simulink model "W06_Tiny_Town_cs"  (R2019a)
settings: Solver=ode5  StartTime=0.0  StopTime=inf  FixedStep=1/20  RelTol=1e-3
PreLoadFcn:
  | mbxruntime.callbacks.PreLoadFcn(bdroot);
PostLoadFcn:
  | mbxruntime.callbacks.PostLoadFcn(bdroot);
InitFcn:
  | mbxruntime.callbacks.InitFcn(bdroot);
StartFcn:
  | mbxruntime.callbacks.StartFcn(bdroot);
StopFcn:
  | mbxruntime.callbacks.StopFcn(bdroot);
model workspace: external: MAT-File .\W06_Tiny_Town_cs_hws.mat (data not in the file)
undefined symbols (not defined in the file or in its folder): DiscIntNeverNeededParam, InitImageOutputDir, mbxruntime, tabledata, W06_Tiny_Town_cs_0347f368afc477f7, W06_Tiny_Town_cs_06d739b3240d4bd1, W06_Tiny_Town_cs_0f8ec0220805dc92, W06_Tiny_Town_cs_158eea2914cd8c14, W06_Tiny_Town_cs_18b17a0c58606dc8, W06_Tiny_Town_cs_19806d8538d6bb90, W06_Tiny_Town_cs_1ceb610c831ebc6c, W06_Tiny_Town_cs_24c71a941f2399ee, W06_Tiny_Town_cs_28d17e17e50ff375, W06_Tiny_Town_cs_29e44574efa0e72f, W06_Tiny_Town_cs_2ebfd9727ae5049f, W06_Tiny_Town_cs_3b9dd96920beca23, W06_Tiny_Town_cs_4a5ba1a10aa72aa4, W06_Tiny_Town_cs_4b7992cae6b11fea, W06_Tiny_Town_cs_4ce1089559374df3, W06_Tiny_Town_cs_4f1eca6f5670696f, W06_Tiny_Town_cs_56de7514e81a64a4, W06_Tiny_Town_cs_5815099e4ab8d5b1, W06_Tiny_Town_cs_59a193f7803a15f8, W06_Tiny_Town_cs_5a93c0b4041e538b, W06_Tiny_Town_cs_5e22ff2291c0d8f8, W06_Tiny_Town_cs_664a4c8dcb6e1d77, W06_Tiny_Town_cs_66e74ff0a825ce8c, W06_Tiny_Town_cs_6f6fc115e33636b9, W06_Tiny_Town_cs_762b24f74e6359cd, W06_Tiny_Town_cs_7e7dfe0ad6d20cde, W06_Tiny_Town_cs_8dbb769f58f1ae22, W06_Tiny_Town_cs_9732a70429881892, W06_Tiny_Town_cs_97e2037932c1d396, W06_Tiny_Town_cs_99e9b9fe56cd6c11, W06_Tiny_Town_cs_9d4b19fadf9db3f5, W06_Tiny_Town_cs_9e5d5712939b904c, W06_Tiny_Town_cs_9fe5ad465f6cdbf3, W06_Tiny_Town_cs_a263437ac60b94d3, W06_Tiny_Town_cs_a313ed4746bdbf42, W06_Tiny_Town_cs_a3bc7bd64557c06d, W06_Tiny_Town_cs_af25170a5cd54ac4, W06_Tiny_Town_cs_b0bfde99f178c69e, W06_Tiny_Town_cs_b828188f0394b7ed, W06_Tiny_Town_cs_b8ac5a8063403724, W06_Tiny_Town_cs_c0c1ce03c301d04b, W06_Tiny_Town_cs_c5d7b9713d9c4410, W06_Tiny_Town_cs_cce5d3f0bd4fe0dd, W06_Tiny_Town_cs_d4161cd6ae7b274e, W06_Tiny_Town_cs_d7f1a2863608ebc5, W06_Tiny_Town_cs_e07aed9c56d02b7c, W06_Tiny_Town_cs_e4fcf49468faab60, W06_Tiny_Town_cs_e81ada3a1b2b4b0f, W06_Tiny_Town_cs_f328760c8f041e3e, W06_Tiny_Town_cs_fbbe35eb7fc27d63, W06_Tiny_Town_cs_fe7173e9daa72ca4, W06_Tiny_Town_cs_Female_Regular_1_Path_pathUniqueID, W06_Tiny_Town_cs_Ford_Focus_Stationwagon_2_Path_pathUniqueID, W06_Tiny_Town_cs_Nissan_Cabstar_Boxtruck_1_Path_pathUniqueID
libraries: PreScanSimulinkLibrary x16, adeye_lib x14, simulink x4, simulink_extras x3, PreScanUsefulBlocks x1
(part 1 of 7)
CloseFcn:
  | mbxruntime.callbacks.CloseFcn(bdroot);
settings Model: Creator=PRESCAN  LastModifiedBy=adeye
settings DataIOCC: LimitDataPoints=on  SaveFormat=Array  SignalLoggingSaveFormat=ModelDataLogs  ReturnWorkspaceOutputs=off
settings OptimizationCC: DefaultParameterBehavior=Inlined  ExpressionDepthLimit=2147483647  InitFltsAndDblsToZero=on  LifeSpan=inf
settings DebuggingCC: SaveWithParameterizedLinksMsg=none  UnderspecifiedInitializationDetection=Classic  MergeDetectMultiDrivingBlocksExec=none  SignalResolutionControl=TryResolveAllWithWarning  MultiTaskDSMMsg=warning  MultiTaskCondExecSysMsg=none  FcnCallInpInsideContextMsg=warning  StateNameClashWarn=warning  SFUnexpectedBacktrackingDiag=warning  SFNoUnconditionalDefaultTransitionDiag=warning  SFExecutionAtInitializationDiag=none  ArithmeticOperatorsInVariantConditions=warning
settings HardwareCC: ProdBitPerPointer=32  ProdBitPerSizeT=32  ProdBitPerPtrDiffT=32  ProdLargestAtomicFloat=None  ProdIntDivRoundTo=Undefined  ProdEndianess=Unspecified  ProdWordSize=32  ProdHWDeviceType=32-bit Generic
settings ModelReferenceCC: UpdateModelReferenceTargets=IfOutOfDate  PropagateSignalLabelsOutOfModel=off
settings SFSimCC: SimUseLocalCustomCode=off  SimParseCustomCode=off
settings SFSimCC: SimCustomHeaderCode=|
  | #include "prescan.h"
  | #include "prescan_platform.h"
  | #include "prescan_aimsunturnindicatorsetter_data.h"
settings RTWCC: RTWUseLocalCustomCode=off
settings CodeAppCC: StateflowObjectComments=on
settings GRTTargetCC: TargetFcnLib=ansi_tfl_tmw.mat  TargetLangStandard=C89/C90 (ANSI)  GeneratePreprocessorConditionals=Disable all  CombineOutputUpdateFcns=off  GRTInterface=on
settings ConfigComp: CovMetricSettings=dw  CovHtmlReporting=on  CovSaveCumulativeToWorkspaceVar=on  CovSaveSingleToWorkspaceVar=on  CovExternalEMLEnable=off  CovSFcnEnable=off

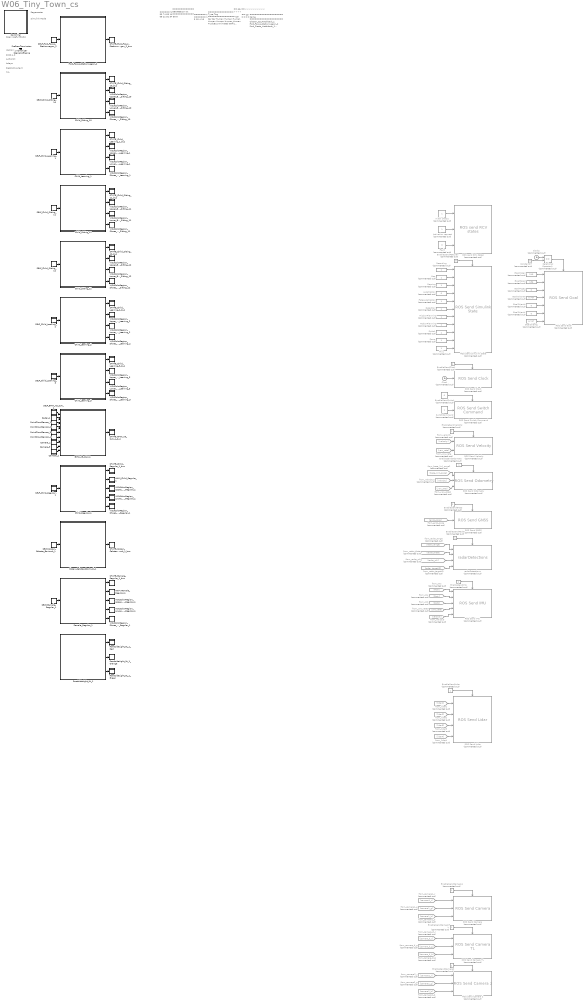
== system W06_Tiny_Town_cs ==
  note: Regenerate
  note: Simulink Mode
  note: Open Useful Blocks
  note: 2020.4.0
  note: Version:
  note: Author(s):
  note: Adeye
  note: Descriptive text:
  note: N.A.
  note: ======
      | Num ID
      | ======
      | 53
      | 74
      | 83
      | 101
      | 102
      | 103
      | 104
      | 67
      | 68
      | 22
      | 52
      | 54
      | 58
      | 8
  note: =============
      | OBU-Beacon ID
      | =============
  note: =======
      | Type ID
      | =======
      | 1
      | 1
      | 1
      | 4
      | 4
      | 4
      | 4
      | 4
      | 4
      | 4
      | 3
      | 15
      | 4
      | 15
  note: ================
      | Type Tag
      | ================
      | Car
      | Car
      | Car
      | Human
      | Human
      | Human
      | Human
      | Human
      | Human
      | Human
      | Truck\Bus
      | Animated traffic sign
      | Human
      | Animated traffic sign
  note: ==
      | SD
      | ==
      | Y
      | Y
      | Y
      | Y
      | Y
      | Y
      | Y
      | Y
      | Y
      | Y
      | Y
      | Y
      | Y
      | Y
  note: ==
      | CD
      | ==
      | N
      | N
      | N
      | N
      | N
      | N
      | N
      | N
      | N
      | N
      | N
      | N
      | N
      | N
  note: ====================
      | Name
      | ====================
      | Citroen_C3_Hatchback_1
      | Ford_Focus_Stationwagon_2
      | Ford_Fiesta_Hatchback_1
      | Child_Sitting_10
      | Child_Leaning_1
      | Child_Sitting_11
      | Child_Sitting_12
      | Child_Leaning_2
      | Child_Leaning_3
      | Child_Regular_1
      | Nissan_Cabstar_Boxtruck_1
      | PedestrianSignal_JP_1
      | Female_Regular_1
      | RoadsideLight_NL_1
  ANIM_Child_Regular_1 : Subsystem  Tag=actuator/AnimationOutport  Priority=0  LoadFcn=load('PreScanAnimActuatorData.mat')  mask(PreScan Sink Block: State Animation){}
      mask help: The Human Animation port allows the human to walk, run or bend
      settings: OpenFcn=open_system([gcb '/Actuator'],'mask')
      mask Help: eval('openHelp(239)')
      mask Display: image(imread('HumanAnimated.jpg'))
  ANIM_Female_Regular_1 : Subsystem  Tag=actuator/AnimationOutport  Priority=0  LoadFcn=load('PreScanAnimActuatorData.mat')  mask(PreScan Sink Block: State Animation){}
      mask help: The Human Animation port allows the human to walk, run or bend
      settings: OpenFcn=open_system([gcb '/Actuator'],'mask')
      mask Help: eval('openHelp(239)')
      mask Display: image(imread('HumanAnimated.jpg'))
  Activation request : Constant  Commented=on  OutDataTypeStr=Inherit: Inherit via back propagation
  BMW_X5_SUV_1 : Subsystem  Tag=WorldObjectSubSystem  InitFcn=UniqueId = '27928';
      mask init:
      | modelPath = GenericModelHelper.getGenericModelFilePath('ModelDepo','Vehicles\BMW_X5\BMW_X5.pgmb','bfeb1c11467705ab888b3011684c848b');imagePath = GenericModelHelper.getCompilationPicture(modelPath, 'BMW_X5_HighPoly.png');
      mask Display: image(imread(imagePath));color('white');text(0, 0, ' ID=21\n')
  Camera_1 : Subsystem  Tag=sensor/Camera/CameraSensor  Priority=30  mask(PreScan Source Block: Camera Sensor){}
      mask help: The Camera Sensor provides a color or monochrome image.
      settings: OpenFcn=open_system([gcb '/Sensor'],'mask')
      mask Help: eval('openHelp(457)')
      mask Display: image(imread('CameraSensor.png'))
  Camera_2 : Subsystem  Tag=sensor/Camera/CameraSensor  Priority=30  mask(PreScan Source Block: Camera Sensor){}
      mask help: The Camera Sensor provides a color or monochrome image.
      settings: OpenFcn=open_system([gcb '/Sensor'],'mask')
      mask Help: eval('openHelp(457)')
      mask Display: image(imread('CameraSensor.png'))
  Camera_tl : Subsystem  Tag=sensor/Camera/CameraSensor  Priority=30  mask(PreScan Source Block: Camera Sensor){}
      mask help: The Camera Sensor provides a color or monochrome image.
      settings: OpenFcn=open_system([gcb '/Sensor'],'mask')
      mask Help: eval('openHelp(457)')
      mask Display: image(imread('CameraSensor.png'))
  Child_Leaning_1 : Subsystem  Tag=WorldObjectSubSystem  InitFcn=UniqueId = '26684';
      mask init:
      | modelPath = GenericModelHelper.getGenericModelFilePath('ModelDepo','Humans\ChildLeaning\Child_Leaning.pgmb','149084199580221ad83bf2ac4272af8c');imagePath = GenericModelHelper.getCompilationPicture(modelPath, 'ChildLeaning.png');
      mask Display: image(imread(imagePath));color('white');text(0, 0, ' ID=102\n')
  Child_Leaning_2 : Subsystem  Tag=WorldObjectSubSystem  InitFcn=UniqueId = '26837';
      mask init: same as W06_Tiny_Town_cs/Child_Leaning_1
      mask Display: image(imread(imagePath));color('white');text(0, 0, ' ID=67\n')
  Child_Leaning_3 : Subsystem  Tag=WorldObjectSubSystem  InitFcn=UniqueId = '26838';
      mask init: same as W06_Tiny_Town_cs/Child_Leaning_1
      mask Display: image(imread(imagePath));color('white');text(0, 0, ' ID=68\n')
  Child_Regular_1 : Subsystem  Tag=WorldObjectSubSystem  InitFcn=UniqueId = '28581';
      mask init:
      | modelPath = GenericModelHelper.getGenericModelFilePath('ModelDepo','Humans\ChildRegular\Child_Regular.pgmb','0405fb6e1c51d7af34e60031bef9e83f');imagePath = GenericModelHelper.getCompilationPicture(modelPath, 'ChildRegular.png');
      mask Display: image(imread(imagePath));color('white');text(0, 0, ' ID=22\n')
  Child_Sitting_10 : Subsystem  Tag=WorldObjectSubSystem  InitFcn=UniqueId = '26683';
      mask init:
      | modelPath = GenericModelHelper.getGenericModelFilePath('ModelDepo','Humans\ChildSitting\Child_Sitting.pgmb','faf3e32d5db0389762af6d34f4b36d2c');imagePath = GenericModelHelper.getCompilationPicture(modelPath, 'ChildSitting.png');
      mask Display: image(imread(imagePath));color('white');text(0, 0, ' ID=101\n')
  Child_Sitting_11 : Subsystem  Tag=WorldObjectSubSystem  InitFcn=UniqueId = '26685';
      mask init: same as W06_Tiny_Town_cs/Child_Sitting_10
      mask Display: image(imread(imagePath));color('white');text(0, 0, ' ID=103\n')
  Child_Sitting_12 : Subsystem  Tag=WorldObjectSubSystem  InitFcn=UniqueId = '26686';
      mask init: same as W06_Tiny_Town_cs/Child_Sitting_10
      mask Display: image(imread(imagePath));color('white');text(0, 0, ' ID=104\n')
  Clock : Clock  Commented=on
  Clock2 : Clock  Commented=on
  Constant27 : Constant  Commented=on  Value=0
  Controller : Subsystem  Description=8A3CD2955739A82C886C20AE3E253D78460D53180EE2C1B14CC08DF75A70BE77  Priority=-1  LoadFcn=load PreScanControllerData  mask(PreScan Simulation Controller){prescanversion='2020.4.0', ModelReferencing=off, TimeStep=1/20, ControlMode=0, PreScanExecutionMode=on, ControllerCount=0, ControllerIndex=0, ControllerOptions=''}
      mask prompts: prescanversion "PreScan Version"; ModelReferencing "Use Model Referencing"; TimeStep "Upload Period [s]"; ControlMode "Control Mode"; PreScanExecutionMode "Execution Mode"; ControllerCount "Controller Count"; ControllerIndex "Controller Index"; ControllerOptions "Controller Options"
      mask help:
      | Please do not remove this block from the compilation sheet,
      | as it connects the model to the PreScan environment.
      mask init:
      | model = bdroot(gcb);
      | ExperimentFile = mbxruntime.findExperimentFile(model,true); %relative path
      | 
      | [d1, d2, d3, prescandata] = prescan_Settings();
      | ModelDepo = fullfile(prescandata,'ModelDepo'); 
      | 
      | RTmode = mbxruntime.getRTMode(model);
      | 
      | SimulationMode = get_param(bdroot,'SimulationMode');
      | if strcmp(SimulationMode, 'rapid-accelerator')
      |     SimulationMode = 'external';
      | end
      | TargetName = get_param(bdroot,'SystemTargetFile');
      settings: ModelCloseFcn=assignin('base',['model_closed_' bdroot],true);
      mask Help: eval('openHelp(812)')
      mask Display: image(imread('prescanlogo.ico'))
  Detection : Constant  Commented=on
  EnableSendCamera1 : Constant  Commented=on  OutDataTypeStr=Inherit: Inherit via back propagation
  EnableSendCamera2 : Constant  Commented=on  OutDataTypeStr=Inherit: Inherit via back propagation
  EnableSendCameraTL : Constant  Commented=on  OutDataTypeStr=Inherit: Inherit via back propagation
  EnableSendClock : Constant  Commented=on  OutDataTypeStr=Inherit: Inherit via back propagation
  EnableSendFeatures : Constant  Commented=on  Value=0  OutDataTypeStr=Inherit: Inherit via back propagation
  EnableSendGNSS : Constant  Commented=on  OutDataTypeStr=Inherit: Inherit via back propagation
  EnableSendIMU : Constant  Commented=on  OutDataTypeStr=Inherit: Inherit via back propagation
  EnableSendLidar : Constant  Commented=on  OutDataTypeStr=Inherit: Inherit via back propagation
  EnableSendOdometry : Constant  Commented=on
  EnableSendRadar : Constant  Commented=on  OutDataTypeStr=Inherit: Inherit via back propagation
  EnableSendSwitch : Constant  Commented=on  Value=0  OutDataTypeStr=Inherit: Inherit via back propagation  SampleTime=0.05
  EnableSendVelocity : Constant  Commented=on  OutDataTypeStr=Inherit: Inherit via back propagation
  FakeLocalization : Constant  Commented=on
  Fault : Constant  Commented=on  Value=0  OutDataTypeStr=Inherit: Inherit via back propagation
  Female_Regular_1 : Subsystem  Tag=WorldObjectSubSystem  InitFcn=UniqueId = '28708';
      mask init:
      | modelPath = GenericModelHelper.getGenericModelFilePath('ModelDepo','Humans\FemaleRegular\Female_Regular.pgmb','a60942a07dc01011c3a5e5a36c910370');imagePath = GenericModelHelper.getCompilationPicture(modelPath, 'FemaleRegular.png');
      mask Display: image(imread(imagePath));color('white');text(0, 0, ' ID=58\n')
  Ford_Focus_Stationwagon_2 : Subsystem  Tag=WorldObjectSubSystem  InitFcn=UniqueId = '26646';
      mask init:
      | modelPath = GenericModelHelper.getGenericModelFilePath('ModelDepo','Vehicles\Ford_Focus_Wagon\Ford_Focus_Wagon.pgmb','daf8bd73c88a9bb5f3f179d705958474');imagePath = GenericModelHelper.getCompilationPicture(modelPath, 'Ford_Focus_Wagon.png');
      mask Display: image(imread(imagePath));color('white');text(0, 0, ' ID=74\n')
  GoalOrientW : Constant  Commented=on  Value=0.707
  GoalOrientX : Constant  Commented=on  Value=0
  GoalOrientY : Constant  Commented=on  Value=0
  GoalOrientZ : Constant  Commented=on  Value=0.707
  GoalPoseX : Constant  Commented=on  Value=249
  GoalPoseY : Constant  Commented=on  Value=136
  GoalPoseZ : Constant  Commented=on  Value=0
  Initial checks : Constant  Commented=on  OutDataTypeStr=Inherit: Inherit via back propagation
  Localization : Constant  Commented=on  Value=0
  Map : Constant  Commented=on
  MissionPlanning : Constant  Commented=on
  MotionPlanning : Constant  Commented=on
  Nissan_Cabstar_Boxtruck_1 : Subsystem  Tag=WorldObjectSubSystem  InitFcn=UniqueId = '28598';
      mask init:
      | modelPath = GenericModelHelper.getGenericModelFilePath('ModelDepo','Vehicles\Nissan_Cabstar\Nissan_Cabstar.pgmb','dd076fdae311093c5436e82e6c23dc23');imagePath = GenericModelHelper.getCompilationPicture(modelPath, 'Nissan_Cabstar_HighPoly.png');
      mask Display: image(imread(imagePath));color('white');text(0, 0, ' ID=52\n')
  PointCloudSensor_1 : Subsystem  Tag=sensor/PointCloudInport  Priority=30  mask(PreScan Source Block: Point Cloud Sensor){}
      mask help: The Point Cloud Sensor provides XYZ positions relative to the sensor
      settings: OpenFcn=open_system([gcb '/Sensor'],'mask')
      mask Help: eval('openHelp(6400)')
      mask Display: image(imread('PointCloudSensorSL.png'))
  PointCloudSensor_2 : Subsystem  Tag=sensor/PointCloudInport  Priority=30  mask(PreScan Source Block: Point Cloud Sensor){}
      mask help: The Point Cloud Sensor provides XYZ positions relative to the sensor
      settings: OpenFcn=open_system([gcb '/Sensor'],'mask')
      mask Help: eval('openHelp(6400)')
      mask Display: image(imread('PointCloudSensorSL.png'))
  PointCloudSensor_3 : Subsystem  Tag=sensor/PointCloudInport  Priority=30  mask(PreScan Source Block: Point Cloud Sensor){}
      mask help: The Point Cloud Sensor provides XYZ positions relative to the sensor
      settings: OpenFcn=open_system([gcb '/Sensor'],'mask')
      mask Help: eval('openHelp(6400)')
      mask Display: image(imread('PointCloudSensorSL.png'))
  PointCloudSensor_4 : Subsystem  Tag=sensor/PointCloudInport  Priority=30  mask(PreScan Source Block: Point Cloud Sensor){}
      mask help: The Point Cloud Sensor provides XYZ positions relative to the sensor
      settings: OpenFcn=open_system([gcb '/Sensor'],'mask')
      mask Help: eval('openHelp(6400)')
      mask Display: image(imread('PointCloudSensorSL.png'))
  PreScanTerminator : Subsystem  Tag=PreScanTerminator  Priority=999  LoadFcn=load PrescanTerminatorData  mask(PreScan Simulation Terminator){TimeStep=1/20}
      mask prompts: TimeStep "Upload Period [s]"
      mask help:
      | Please do not remove this block from the compilation sheet as it
      | connects the model to the PreScan environment.
      mask Help: eval('openHelp(812)')
      mask Display: image(imread('prescanlogo.ico'))
  ROS Send Camera : adeye_lib/ROS Send Camera  Commented=on  SystemSampleTime=-1
  ROS Send Camera 2 : adeye_lib/ROS Send Camera 2  Commented=on  SystemSampleTime=-1
  ROS Send Camera TL : adeye_lib/ROS Send Camera TL  Commented=on  SystemSampleTime=-1
  ROS Send Clock : adeye_lib/ROS Send Clock  Commented=on  SystemSampleTime=-1
  ROS Send GNSS : adeye_lib/ROS Send GNSS  Commented=on  SystemSampleTime=-1
  ROS Send Goal : adeye_lib/ROS Send Goal  Commented=on  SystemSampleTime=-1
  ROS Send IMU : adeye_lib/ROS Send IMU  Commented=on  SystemSampleTime=-1
  ROS Send Lidar : adeye_lib/ROS Send Lidar  Commented=on  SystemSampleTime=-1
  ROS Send Odometry : adeye_lib/ROS Send Odometry  Commented=on  SystemSampleTime=-1
  ROS Send Simulink State : adeye_lib/ROS Send Simulink State  Commented=on  SystemSampleTime=-1
  ROS Send Switch Command : adeye_lib/ROS Send Switch Command  Commented=on  SystemSampleTime=-1
  ROS Send Velocity : adeye_lib/ROS Send Velocity  Commented=on  SystemSampleTime=-1
  ROS send RCV states : adeye_lib/ROS send RCV states  Commented=on  SystemSampleTime=-1
  Radar_1 : Subsystem  Tag=sensor/Radar  Priority=30  LoadFcn=load('PrescanScannerSensorData.mat');load('PrescanScannerSensorMessage.mat')  mask(PreScan Source Block: Radar Sensor){}
      mask help:
      | The Radar Sensor is a detailed sensor based on a physical radar
      | model that includes Antenna GAIN Maps (AGM) and atmospheric
      | attenuation.
      |
      | For more information, please click Help.
      settings: OpenFcn=open_system([gcb '/Sensor'],'mask')
      mask Help: eval('openHelp(1464)')
      mask Display: image(imread('Radar.png'))
  Recording : Constant  Commented=on
  Relational Operator1 : RelationalOperator  Commented=on  Operator===  OutDataTypeStr=boolean  RndMeth=Simplest
  RoadsideLight_NL_1 : Subsystem  Tag=WorldObjectSubSystem  InitFcn=UniqueId = '31564';
      mask init:
      | modelPath = GenericModelHelper.getGenericModelFilePath('ModelDepo','AnimatedElements\TrafficLight_NL\Roadside\Roadside_NL.pgmb','2000fba5e1a6d0fba32e88146243c3cb');imagePath = GenericModelHelper.getCompilationPicture(modelPath, 'Roadside_NL.png');
      mask Display: image(imread(imagePath));color('white');text(0, 0, ' ID=8\n')
  RoadsideLight_NL_1_Green : Subsystem  Tag=actuator/Green  Priority=0  LoadFcn=load('PreScanVisuLightActuatorData');load('PrescanRPYData');load('PrescanXYZData');load('PreScanRGBData')  mask(PreScan Sink Block: VisuActiveLight){}
      mask help:
      | The VisuActiveLight block provides a way for detailed animation of Light Sources, such as the indicator, brake, fog and main lights of a vehicle, or a light post.
      |
      | For more information, please click Help.
      settings: OpenFcn=open_system([gcb '/Actuator'],'mask')
      mask Help: eval('openHelp(209)')
      mask Display: image(imread('HeadLight.png'))
  RoadsideLight_NL_1_Orange : Subsystem  Tag=actuator/Orange  Priority=0  LoadFcn=load('PreScanVisuLightActuatorData');load('PrescanRPYData');load('PrescanXYZData');load('PreScanRGBData')  mask(PreScan Sink Block: VisuActiveLight){}
      mask help:
      | The VisuActiveLight block provides a way for detailed animation of Light Sources, such as the indicator, brake, fog and main lights of a vehicle, or a light post.
      |
      | For more information, please click Help.
      settings: OpenFcn=open_system([gcb '/Actuator'],'mask')
      mask Help: eval('openHelp(209)')
      mask Display: image(imread('HeadLight.png'))
  RoadsideLight_NL_1_Red : Subsystem  Tag=actuator/Red  Priority=0  LoadFcn=load('PreScanVisuLightActuatorData');load('PrescanRPYData');load('PrescanXYZData');load('PreScanRGBData')  mask(PreScan Sink Block: VisuActiveLight){}
      mask help:
      | The VisuActiveLight block provides a way for detailed animation of Light Sources, such as the indicator, brake, fog and main lights of a vehicle, or a light post.
      |
      | For more information, please click Help.
      settings: OpenFcn=open_system([gcb '/Actuator'],'mask')
      mask Help: eval('openHelp(209)')
      mask Display: image(imread('HeadLight.png'))
  Rviz : Constant  Commented=on
  SELF_BMW_X5_SUV_1 : Subsystem  Tag=sensor/SelfPort  Priority=30  LoadFcn=load('PreScanSelfSensorData.mat')  mask(PreScan Source Block: SELF){}
      mask help:
      | The SELF port shows (state) information of the actor itself. The outputs are position in the experiment's axis system and the GPS coordinates, and the object's absolute velocity and compass heading.
      |
      | For more information, please click Help.
      settings: OpenFcn=open_system([gcb '/Sensor'],'mask')
      mask Help: eval('openHelp(462)')
      mask Display: image(imread('GPS.png'))
  SELF_Child_Leaning_1 : Subsystem  Tag=sensor/SelfPort  Priority=30  LoadFcn=load('PreScanSelfSensorData.mat')  mask(PreScan Source Block: SELF){}
      mask help:
      | The SELF port shows (state) information of the actor itself. The outputs are position in the experiment's axis system and the GPS coordinates, and the object's absolute velocity and compass heading.
      |
      | For more information, please click Help.
      settings: OpenFcn=open_system([gcb '/Sensor'],'mask')
      mask Help: eval('openHelp(462)')
      mask Display: image(imread('GPS.png'))
  SELF_Child_Leaning_2 : Subsystem  Tag=sensor/SelfPort  Priority=30  LoadFcn=load('PreScanSelfSensorData.mat')  mask(PreScan Source Block: SELF){}
      mask help:
      | The SELF port shows (state) information of the actor itself. The outputs are position in the experiment's axis system and the GPS coordinates, and the object's absolute velocity and compass heading.
      |
      | For more information, please click Help.
      settings: OpenFcn=open_system([gcb '/Sensor'],'mask')
      mask Help: eval('openHelp(462)')
      mask Display: image(imread('GPS.png'))
  SELF_Child_Leaning_3 : Subsystem  Tag=sensor/SelfPort  Priority=30  LoadFcn=load('PreScanSelfSensorData.mat')  mask(PreScan Source Block: SELF){}
      mask help:
      | The SELF port shows (state) information of the actor itself. The outputs are position in the experiment's axis system and the GPS coordinates, and the object's absolute velocity and compass heading.
      |
      | For more information, please click Help.
      settings: OpenFcn=open_system([gcb '/Sensor'],'mask')
      mask Help: eval('openHelp(462)')
      mask Display: image(imread('GPS.png'))
  SELF_Child_Regular_1 : Subsystem  Tag=sensor/SelfPort  Priority=30  LoadFcn=load('PreScanSelfSensorData.mat')  mask(PreScan Source Block: SELF){}
      mask help:
      | The SELF port shows (state) information of the actor itself. The outputs are position in the experiment's axis system and the GPS coordinates, and the object's absolute velocity and compass heading.
      |
      | For more information, please click Help.
      settings: OpenFcn=open_system([gcb '/Sensor'],'mask')
      mask Help: eval('openHelp(462)')
      mask Display: image(imread('GPS.png'))
  SELF_Child_Sitting_10 : Subsystem  Tag=sensor/SelfPort  Priority=30  LoadFcn=load('PreScanSelfSensorData.mat')  mask(PreScan Source Block: SELF){}
      mask help:
      | The SELF port shows (state) information of the actor itself. The outputs are position in the experiment's axis system and the GPS coordinates, and the object's absolute velocity and compass heading.
      |
      | For more information, please click Help.
      settings: OpenFcn=open_system([gcb '/Sensor'],'mask')
      mask Help: eval('openHelp(462)')
      mask Display: image(imread('GPS.png'))
  SELF_Child_Sitting_11 : Subsystem  Tag=sensor/SelfPort  Priority=30  LoadFcn=load('PreScanSelfSensorData.mat')  mask(PreScan Source Block: SELF){}
      mask help:
      | The SELF port shows (state) information of the actor itself. The outputs are position in the experiment's axis system and the GPS coordinates, and the object's absolute velocity and compass heading.
      |
      | For more information, please click Help.
      settings: OpenFcn=open_system([gcb '/Sensor'],'mask')
      mask Help: eval('openHelp(462)')
      mask Display: image(imread('GPS.png'))
  SELF_Child_Sitting_12 : Subsystem  Tag=sensor/SelfPort  Priority=30  LoadFcn=load('PreScanSelfSensorData.mat')  mask(PreScan Source Block: SELF){}
      mask help:
      | The SELF port shows (state) information of the actor itself. The outputs are position in the experiment's axis system and the GPS coordinates, and the object's absolute velocity and compass heading.
      |
      | For more information, please click Help.
      settings: OpenFcn=open_system([gcb '/Sensor'],'mask')
      mask Help: eval('openHelp(462)')
      mask Display: image(imread('GPS.png'))
  SELF_Female_Regular_1 : Subsystem  Tag=sensor/SelfPort  Priority=30  LoadFcn=load('PreScanSelfSensorData.mat')  mask(PreScan Source Block: SELF){}
      mask help:
      | The SELF port shows (state) information of the actor itself. The outputs are position in the experiment's axis system and the GPS coordinates, and the object's absolute velocity and compass heading.
      |
      | For more information, please click Help.
      settings: OpenFcn=open_system([gcb '/Sensor'],'mask')
      mask Help: eval('openHelp(462)')
      mask Display: image(imread('GPS.png'))
  SELF_Ford_Focus_Stationwagon_2 : Subsystem  Tag=sensor/SelfPort  Priority=30  LoadFcn=load('PreScanSelfSensorData.mat')  mask(PreScan Source Block: SELF){}
      mask help:
      | The SELF port shows (state) information of the actor itself. The outputs are position in the experiment's axis system and the GPS coordinates, and the object's absolute velocity and compass heading.
      |
      | For more information, please click Help.
      settings: OpenFcn=open_system([gcb '/Sensor'],'mask')
      mask Help: eval('openHelp(462)')
      mask Display: image(imread('GPS.png'))
  SELF_Nissan_Cabstar_Boxtruck_1 : Subsystem  Tag=sensor/SelfPort  Priority=30  LoadFcn=load('PreScanSelfSensorData.mat')  mask(PreScan Source Block: SELF){}
      mask help:
      | The SELF port shows (state) information of the actor itself. The outputs are position in the experiment's axis system and the GPS coordinates, and the object's absolute velocity and compass heading.
      |
      | For more information, please click Help.
      settings: OpenFcn=open_system([gcb '/Sensor'],'mask')
      mask Help: eval('openHelp(462)')
      mask Display: image(imread('GPS.png'))
  STATE_BMW_X5_SUV_1_bus : Subsystem  Tag=actuator/StatePort  Priority=0  LoadFcn=load('PreScanStateActuatorData.mat')  mask(PreScan Sink Block: State){}
      mask help:
      | The Actor State contains a vector signal of size (9x1), containing the following signals:
      |
      | -  Position    	(x,y,z)             	[m]
      | -  Velocity    	(vx,vy,vz)         	[m/s]
      | -  Angles       	(Roll, Pitch, Yaw)	[rad]
      |
      | The Actor state is defined in the global axis system.
      | The state is superponed on the Initial position defined in the GUI.
      |
      | For more information, please click Help.
      settings: OpenFcn=open_system([gcb '/Actuator'],'mask')
      mask Help: eval('openHelp(222)')
      mask Display: image(imread('State.png'))
  STATE_Child_Leaning_1_bus : Subsystem  Tag=actuator/StatePort  Priority=0  LoadFcn=load('PreScanStateActuatorData.mat')  mask(PreScan Sink Block: State){}
      mask help:
      | The Actor State contains a vector signal of size (9x1), containing the following signals:
      |
      | -  Position    	(x,y,z)             	[m]
      | -  Velocity    	(vx,vy,vz)         	[m/s]
      | -  Angles       	(Roll, Pitch, Yaw)	[rad]
      |
      | The Actor state is defined in the global axis system.
      | The state is superponed on the Initial position defined in the GUI.
      |
      | For more information, please click Help.
      settings: OpenFcn=open_system([gcb '/Actuator'],'mask')
      mask Help: eval('openHelp(222)')
      mask Display: image(imread('State.png'))
  STATE_Child_Leaning_2_bus : Subsystem  Tag=actuator/StatePort  Priority=0  LoadFcn=load('PreScanStateActuatorData.mat')  mask(PreScan Sink Block: State){}
      mask help:
      | The Actor State contains a vector signal of size (9x1), containing the following signals:
      |
      | -  Position    	(x,y,z)             	[m]
      | -  Velocity    	(vx,vy,vz)         	[m/s]
      | -  Angles       	(Roll, Pitch, Yaw)	[rad]
      |
      | The Actor state is defined in the global axis system.
      | The state is superponed on the Initial position defined in the GUI.
      |
      | For more information, please click Help.
      settings: OpenFcn=open_system([gcb '/Actuator'],'mask')
      mask Help: eval('openHelp(222)')
      mask Display: image(imread('State.png'))
  STATE_Child_Leaning_3_bus : Subsystem  Tag=actuator/StatePort  Priority=0  LoadFcn=load('PreScanStateActuatorData.mat')  mask(PreScan Sink Block: State){}
      mask help:
      | The Actor State contains a vector signal of size (9x1), containing the following signals:
      |
      | -  Position    	(x,y,z)             	[m]
      | -  Velocity    	(vx,vy,vz)         	[m/s]
      | -  Angles       	(Roll, Pitch, Yaw)	[rad]
      |
      | The Actor state is defined in the global axis system.
      | The state is superponed on the Initial position defined in the GUI.
      |
      | For more information, please click Help.
      settings: OpenFcn=open_system([gcb '/Actuator'],'mask')
      mask Help: eval('openHelp(222)')
      mask Display: image(imread('State.png'))
  STATE_Child_Regular_1_bus : Subsystem  Tag=actuator/StatePort  Priority=0  LoadFcn=load('PreScanStateActuatorData.mat')  mask(PreScan Sink Block: State){}
      mask help:
      | The Actor State contains a vector signal of size (9x1), containing the following signals:
      |
      | -  Position    	(x,y,z)             	[m]
      | -  Velocity    	(vx,vy,vz)         	[m/s]
      | -  Angles       	(Roll, Pitch, Yaw)	[rad]
      |
      | The Actor state is defined in the global axis system.
      | The state is superponed on the Initial position defined in the GUI.
      |
      | For more information, please click Help.
      settings: OpenFcn=open_system([gcb '/Actuator'],'mask')
      mask Help: eval('openHelp(222)')
      mask Display: image(imread('State.png'))
  STATE_Child_Sitting_10_bus : Subsystem  Tag=actuator/StatePort  Priority=0  LoadFcn=load('PreScanStateActuatorData.mat')  mask(PreScan Sink Block: State){}
      mask help:
      | The Actor State contains a vector signal of size (9x1), containing the following signals:
      |
      | -  Position    	(x,y,z)             	[m]
      | -  Velocity    	(vx,vy,vz)         	[m/s]
      | -  Angles       	(Roll, Pitch, Yaw)	[rad]
      |
      | The Actor state is defined in the global axis system.
      | The state is superponed on the Initial position defined in the GUI.
      |
      | For more information, please click Help.
      settings: OpenFcn=open_system([gcb '/Actuator'],'mask')
      mask Help: eval('openHelp(222)')
      mask Display: image(imread('State.png'))
  STATE_Child_Sitting_11_bus : Subsystem  Tag=actuator/StatePort  Priority=0  LoadFcn=load('PreScanStateActuatorData.mat')  mask(PreScan Sink Block: State){}
      mask help:
      | The Actor State contains a vector signal of size (9x1), containing the following signals:
      |
      | -  Position    	(x,y,z)             	[m]
      | -  Velocity    	(vx,vy,vz)         	[m/s]
      | -  Angles       	(Roll, Pitch, Yaw)	[rad]
      |
      | The Actor state is defined in the global axis system.
      | The state is superponed on the Initial position defined in the GUI.
      |
      | For more information, please click Help.
      settings: OpenFcn=open_system([gcb '/Actuator'],'mask')
      mask Help: eval('openHelp(222)')
      mask Display: image(imread('State.png'))
  STATE_Child_Sitting_12_bus : Subsystem  Tag=actuator/StatePort  Priority=0  LoadFcn=load('PreScanStateActuatorData.mat')  mask(PreScan Sink Block: State){}
      mask help:
      | The Actor State contains a vector signal of size (9x1), containing the following signals:
      |
      | -  Position    	(x,y,z)             	[m]
      | -  Velocity    	(vx,vy,vz)         	[m/s]
      | -  Angles       	(Roll, Pitch, Yaw)	[rad]
      |
      | The Actor state is defined in the global axis system.
      | The state is superponed on the Initial position defined in the GUI.
      |
      | For more information, please click Help.
      settings: OpenFcn=open_system([gcb '/Actuator'],'mask')
      mask Help: eval('openHelp(222)')
      mask Display: image(imread('State.png'))
  STATE_Female_Regular_1_bus : Subsystem  Tag=actuator/StatePort  Priority=0  LoadFcn=load('PreScanStateActuatorData.mat')  mask(PreScan Sink Block: State){}
      mask help:
      | The Actor State contains a vector signal of size (9x1), containing the following signals:
      |
      | -  Position    	(x,y,z)             	[m]
      | -  Velocity    	(vx,vy,vz)         	[m/s]
      | -  Angles       	(Roll, Pitch, Yaw)	[rad]
      |
      | The Actor state is defined in the global axis system.
      | The state is superponed on the Initial position defined in the GUI.
      |
      | For more information, please click Help.
      settings: OpenFcn=open_system([gcb '/Actuator'],'mask')
      mask Help: eval('openHelp(222)')
      mask Display: image(imread('State.png'))
  STATE_Ford_Focus_Stationwagon_2_bus : Subsystem  Tag=actuator/StatePort  Priority=0  LoadFcn=load('PreScanStateActuatorData.mat')  mask(PreScan Sink Block: State){}
      mask help:
      | The Actor State contains a vector signal of size (9x1), containing the following signals:
      |
      | -  Position    	(x,y,z)             	[m]
      | -  Velocity    	(vx,vy,vz)         	[m/s]
      | -  Angles       	(Roll, Pitch, Yaw)	[rad]
      |
      | The Actor state is defined in the global axis system.
      | The state is superponed on the Initial position defined in the GUI.
      |
      | For more information, please click Help.
      settings: OpenFcn=open_system([gcb '/Actuator'],'mask')
      mask Help: eval('openHelp(222)')
      mask Display: image(imread('State.png'))
  STATE_Nissan_Cabstar_Boxtruck_1_bus : Subsystem  Tag=actuator/StatePort  Priority=0  LoadFcn=load('PreScanStateActuatorData.mat')  mask(PreScan Sink Block: State){}
      mask help:
      | The Actor State contains a vector signal of size (9x1), containing the following signals:
      |
      | -  Position    	(x,y,z)             	[m]
      | -  Velocity    	(vx,vy,vz)         	[m/s]
      | -  Angles       	(Roll, Pitch, Yaw)	[rad]
      |
      | The Actor state is defined in the global axis system.
      | The state is superponed on the Initial position defined in the GUI.
      |
      | For more information, please click Help.
      settings: OpenFcn=open_system([gcb '/Actuator'],'mask')
      mask Help: eval('openHelp(222)')
      mask Display: image(imread('State.png'))
  ScenarioEngine : Subsystem  Tag=PreScanOpenScenarioBlock  Priority=10  LoadFcn=load PrescanSynchronizeData  mask(PreScan Simulation Core Block){TimeStep=1/20}
      mask prompts: TimeStep "Timestep [s]"
      mask help:
      | Please do not remove this block from the PreScan compilation sheet,
      | as it contains essential configuration parameters for a PreScan simulation.
      settings: DeleteFcn=PreScanBlockDeleteFcn;
      mask Display: image(imread('prescanlogo.ico'))
  Sensing : Constant  Commented=on
  Ssmp : Constant  Commented=on
  Switch : Constant  Commented=on
  SwitchCommand : Constant  Commented=on  OutDataTypeStr=Inherit: Inherit via back propagation  SampleTime=0.05
  Synchronizer : Subsystem  Tag=PreScanSynchronizer  Priority=20  LoadFcn=load PrescanSynchronizeData  mask(PreScan Simulation Core Block){TimeStep=1/20}
      mask prompts: TimeStep "Timestep [s]"
      mask help:
      | Please do not remove this block from the PreScan compilation sheet,
      | as it contains essential configuration parameters for a PreScan simulation.
      settings: DeleteFcn=PreScanBlockDeleteFcn;
      mask Display: image(imread('prescanlogo.ico'))
  VISUColorRegion_Lower_Body_Child_Leaning_1 : Subsystem  Tag=actuator/ColorRegion  Priority=0  LoadFcn=load('PrescanColorData')  mask(PreScan Sink Block: VisuTextureColor){}
      mask help:
      | The VisuTextureColor block provides a way to adapt the color of a vehicle.
      |
      | For more information, please click Help.
      settings: OpenFcn=open_system([gcb '/Actuator'],'mask')
      mask Help: eval('openHelp(230)')
      mask Display: image(imread('TextureColor.png'))
  VISUColorRegion_Lower_Body_Child_Leaning_2 : Subsystem  Tag=actuator/ColorRegion  Priority=0  LoadFcn=load('PrescanColorData')  mask(PreScan Sink Block: VisuTextureColor){}
      mask help:
      | The VisuTextureColor block provides a way to adapt the color of a vehicle.
      |
      | For more information, please click Help.
      settings: OpenFcn=open_system([gcb '/Actuator'],'mask')
      mask Help: eval('openHelp(230)')
      mask Display: image(imread('TextureColor.png'))
  VISUColorRegion_Lower_Body_Child_Leaning_3 : Subsystem  Tag=actuator/ColorRegion  Priority=0  LoadFcn=load('PrescanColorData')  mask(PreScan Sink Block: VisuTextureColor){}
      mask help:
      | The VisuTextureColor block provides a way to adapt the color of a vehicle.
      |
      | For more information, please click Help.
      settings: OpenFcn=open_system([gcb '/Actuator'],'mask')
      mask Help: eval('openHelp(230)')
      mask Display: image(imread('TextureColor.png'))
  VISUColorRegion_Lower_Body_Child_Regular_1 : Subsystem  Tag=actuator/ColorRegion  Priority=0  LoadFcn=load('PrescanColorData')  mask(PreScan Sink Block: VisuTextureColor){}
      mask help:
      | The VisuTextureColor block provides a way to adapt the color of a vehicle.
      |
      | For more information, please click Help.
      settings: OpenFcn=open_system([gcb '/Actuator'],'mask')
      mask Help: eval('openHelp(230)')
      mask Display: image(imread('TextureColor.png'))
  VISUColorRegion_Lower_Body_Child_Sitting_10 : Subsystem  Tag=actuator/ColorRegion  Priority=0  LoadFcn=load('PrescanColorData')  mask(PreScan Sink Block: VisuTextureColor){}
      mask help:
      | The VisuTextureColor block provides a way to adapt the color of a vehicle.
      |
      | For more information, please click Help.
      settings: OpenFcn=open_system([gcb '/Actuator'],'mask')
      mask Help: eval('openHelp(230)')
      mask Display: image(imread('TextureColor.png'))
  VISUColorRegion_Lower_Body_Child_Sitting_11 : Subsystem  Tag=actuator/ColorRegion  Priority=0  LoadFcn=load('PrescanColorData')  mask(PreScan Sink Block: VisuTextureColor){}
      mask help:
      | The VisuTextureColor block provides a way to adapt the color of a vehicle.
      |
      | For more information, please click Help.
      settings: OpenFcn=open_system([gcb '/Actuator'],'mask')
      mask Help: eval('openHelp(230)')
      mask Display: image(imread('TextureColor.png'))
  VISUColorRegion_Lower_Body_Child_Sitting_12 : Subsystem  Tag=actuator/ColorRegion  Priority=0  LoadFcn=load('PrescanColorData')  mask(PreScan Sink Block: VisuTextureColor){}
      mask help:
      | The VisuTextureColor block provides a way to adapt the color of a vehicle.
      |
      | For more information, please click Help.
      settings: OpenFcn=open_system([gcb '/Actuator'],'mask')
      mask Help: eval('openHelp(230)')
      mask Display: image(imread('TextureColor.png'))
  VISUColorRegion_Lower_Body_Female_Regular_1 : Subsystem  Tag=actuator/ColorRegion  Priority=0  LoadFcn=load('PrescanColorData')  mask(PreScan Sink Block: VisuTextureColor){}
      mask help:
      | The VisuTextureColor block provides a way to adapt the color of a vehicle.
      |
      | For more information, please click Help.
      settings: OpenFcn=open_system([gcb '/Actuator'],'mask')
      mask Help: eval('openHelp(230)')
      mask Display: image(imread('TextureColor.png'))
  VISUColorRegion_Shoes_Child_Leaning_1 : Subsystem  Tag=actuator/ColorRegion  Priority=0  LoadFcn=load('PrescanColorData')  mask(PreScan Sink Block: VisuTextureColor){}
      mask help:
      | The VisuTextureColor block provides a way to adapt the color of a vehicle.
      |
      | For more information, please click Help.
      settings: OpenFcn=open_system([gcb '/Actuator'],'mask')
      mask Help: eval('openHelp(230)')
      mask Display: image(imread('TextureColor.png'))
  VISUColorRegion_Shoes_Child_Leaning_2 : Subsystem  Tag=actuator/ColorRegion  Priority=0  LoadFcn=load('PrescanColorData')  mask(PreScan Sink Block: VisuTextureColor){}
      mask help:
      | The VisuTextureColor block provides a way to adapt the color of a vehicle.
      |
      | For more information, please click Help.
      settings: OpenFcn=open_system([gcb '/Actuator'],'mask')
      mask Help: eval('openHelp(230)')
      mask Display: image(imread('TextureColor.png'))
  VISUColorRegion_Shoes_Child_Leaning_3 : Subsystem  Tag=actuator/ColorRegion  Priority=0  LoadFcn=load('PrescanColorData')  mask(PreScan Sink Block: VisuTextureColor){}
      mask help:
      | The VisuTextureColor block provides a way to adapt the color of a vehicle.
      |
      | For more information, please click Help.
      settings: OpenFcn=open_system([gcb '/Actuator'],'mask')
      mask Help: eval('openHelp(230)')
      mask Display: image(imread('TextureColor.png'))
  VISUColorRegion_Shoes_Child_Regular_1 : Subsystem  Tag=actuator/ColorRegion  Priority=0  LoadFcn=load('PrescanColorData')  mask(PreScan Sink Block: VisuTextureColor){}
      mask help:
      | The VisuTextureColor block provides a way to adapt the color of a vehicle.
      |
      | For more information, please click Help.
      settings: OpenFcn=open_system([gcb '/Actuator'],'mask')
      mask Help: eval('openHelp(230)')
      mask Display: image(imread('TextureColor.png'))
  VISUColorRegion_Shoes_Child_Sitting_10 : Subsystem  Tag=actuator/ColorRegion  Priority=0  LoadFcn=load('PrescanColorData')  mask(PreScan Sink Block: VisuTextureColor){}
      mask help:
      | The VisuTextureColor block provides a way to adapt the color of a vehicle.
      |
      | For more information, please click Help.
      settings: OpenFcn=open_system([gcb '/Actuator'],'mask')
      mask Help: eval('openHelp(230)')
      mask Display: image(imread('TextureColor.png'))
  VISUColorRegion_Shoes_Child_Sitting_11 : Subsystem  Tag=actuator/ColorRegion  Priority=0  LoadFcn=load('PrescanColorData')  mask(PreScan Sink Block: VisuTextureColor){}
      mask help:
      | The VisuTextureColor block provides a way to adapt the color of a vehicle.
      |
      | For more information, please click Help.
      settings: OpenFcn=open_system([gcb '/Actuator'],'mask')
      mask Help: eval('openHelp(230)')
      mask Display: image(imread('TextureColor.png'))
  VISUColorRegion_Shoes_Child_Sitting_12 : Subsystem  Tag=actuator/ColorRegion  Priority=0  LoadFcn=load('PrescanColorData')  mask(PreScan Sink Block: VisuTextureColor){}
      mask help:
      | The VisuTextureColor block provides a way to adapt the color of a vehicle.
      |
      | For more information, please click Help.
      settings: OpenFcn=open_system([gcb '/Actuator'],'mask')
      mask Help: eval('openHelp(230)')
      mask Display: image(imread('TextureColor.png'))
  VISUColorRegion_Shoes_Female_Regular_1 : Subsystem  Tag=actuator/ColorRegion  Priority=0  LoadFcn=load('PrescanColorData')  mask(PreScan Sink Block: VisuTextureColor){}
      mask help:
      | The VisuTextureColor block provides a way to adapt the color of a vehicle.
      |
      | For more information, please click Help.
      settings: OpenFcn=open_system([gcb '/Actuator'],'mask')
      mask Help: eval('openHelp(230)')
      mask Display: image(imread('TextureColor.png'))
  VISUColorRegion_Upper_Body_Child_Leaning_1 : Subsystem  Tag=actuator/ColorRegion  Priority=0  LoadFcn=load('PrescanColorData')  mask(PreScan Sink Block: VisuTextureColor){}
      mask help:
      | The VisuTextureColor block provides a way to adapt the color of a vehicle.
      |
      | For more information, please click Help.
      settings: OpenFcn=open_system([gcb '/Actuator'],'mask')
      mask Help: eval('openHelp(230)')
      mask Display: image(imread('TextureColor.png'))
  VISUColorRegion_Upper_Body_Child_Leaning_2 : Subsystem  Tag=actuator/ColorRegion  Priority=0  LoadFcn=load('PrescanColorData')  mask(PreScan Sink Block: VisuTextureColor){}
      mask help:
      | The VisuTextureColor block provides a way to adapt the color of a vehicle.
      |
      | For more information, please click Help.
      settings: OpenFcn=open_system([gcb '/Actuator'],'mask')
      mask Help: eval('openHelp(230)')
      mask Display: image(imread('TextureColor.png'))
  VISUColorRegion_Upper_Body_Child_Leaning_3 : Subsystem  Tag=actuator/ColorRegion  Priority=0  LoadFcn=load('PrescanColorData')  mask(PreScan Sink Block: VisuTextureColor){}
      mask help:
      | The VisuTextureColor block provides a way to adapt the color of a vehicle.
      |
      | For more information, please click Help.
      settings: OpenFcn=open_system([gcb '/Actuator'],'mask')
      mask Help: eval('openHelp(230)')
      mask Display: image(imread('TextureColor.png'))
  VISUColorRegion_Upper_Body_Child_Regular_1 : Subsystem  Tag=actuator/ColorRegion  Priority=0  LoadFcn=load('PrescanColorData')  mask(PreScan Sink Block: VisuTextureColor){}
      mask help:
      | The VisuTextureColor block provides a way to adapt the color of a vehicle.
      |
      | For more information, please click Help.
      settings: OpenFcn=open_system([gcb '/Actuator'],'mask')
      mask Help: eval('openHelp(230)')
      mask Display: image(imread('TextureColor.png'))
  VISUColorRegion_Upper_Body_Child_Sitting_10 : Subsystem  Tag=actuator/ColorRegion  Priority=0  LoadFcn=load('PrescanColorData')  mask(PreScan Sink Block: VisuTextureColor){}
      mask help:
      | The VisuTextureColor block provides a way to adapt the color of a vehicle.
      |
      | For more information, please click Help.
      settings: OpenFcn=open_system([gcb '/Actuator'],'mask')
      mask Help: eval('openHelp(230)')
      mask Display: image(imread('TextureColor.png'))
  VISUColorRegion_Upper_Body_Child_Sitting_11 : Subsystem  Tag=actuator/ColorRegion  Priority=0  LoadFcn=load('PrescanColorData')  mask(PreScan Sink Block: VisuTextureColor){}
      mask help:
      | The VisuTextureColor block provides a way to adapt the color of a vehicle.
      |
      | For more information, please click Help.
      settings: OpenFcn=open_system([gcb '/Actuator'],'mask')
      mask Help: eval('openHelp(230)')
      mask Display: image(imread('TextureColor.png'))
  VISUColorRegion_Upper_Body_Child_Sitting_12 : Subsystem  Tag=actuator/ColorRegion  Priority=0  LoadFcn=load('PrescanColorData')  mask(PreScan Sink Block: VisuTextureColor){}
      mask help:
      | The VisuTextureColor block provides a way to adapt the color of a vehicle.
      |
      | For more information, please click Help.
      settings: OpenFcn=open_system([gcb '/Actuator'],'mask')
      mask Help: eval('openHelp(230)')
      mask Display: image(imread('TextureColor.png'))
  VISUColorRegion_Upper_Body_Female_Regular_1 : Subsystem  Tag=actuator/ColorRegion  Priority=0  LoadFcn=load('PrescanColorData')  mask(PreScan Sink Block: VisuTextureColor){}
      mask help:
      | The VisuTextureColor block provides a way to adapt the color of a vehicle.
      |
      | For more information, please click Help.
      settings: OpenFcn=open_system([gcb '/Actuator'],'mask')
      mask Help: eval('openHelp(230)')
      mask Display: image(imread('TextureColor.png'))
  from_base_link_pose2 : From  Commented=on  GotoTag=base_link_pose
  from_camera1_b : From  Commented=on  GotoTag=camera1_b
  from_camera1_g : From  Commented=on  GotoTag=camera1_g
  from_camera1_r : From  Commented=on  GotoTag=camera1_r
  from_camera2_b : From  Commented=on  GotoTag=camera2_b
  from_camera2_g : From  Commented=on  GotoTag=camera2_g
  from_camera2_r : From  Commented=on  GotoTag=camera2_r
  from_camera_tl_b : From  Commented=on  GotoTag=camera_tl_b
  from_camera_tl_g : From  Commented=on  GotoTag=camera_tl_g
  from_camera_tl_r : From  Commented=on  GotoTag=camera_tl_r
  from_gnss_pose : From  Commented=on  GotoTag=gnss_pose
  from_lidar1 : From  Commented=on  GotoTag=lidar1
  from_lidar2 : From  Commented=on  GotoTag=lidar2
  from_lidar3 : From  Commented=on  GotoTag=lidar3
  from_lidar4 : From  Commented=on  GotoTag=lidar4
  from_radar_phi : From  Commented=on  GotoTag=radar_phi
  from_radar_range : From  Commented=on  GotoTag=radar_range
  from_radar_targetID : From  Commented=on  GotoTag=radar_targetID
  from_radar_theta : From  Commented=on  GotoTag=radar_theta
  from_rotx : From  Commented=on  GotoTag=Rotx
  from_roty : From  Commented=on  GotoTag=Roty
  from_rotz : From  Commented=on  GotoTag=Rotz
  from_velicty3 : From  Commented=on  GotoTag=velocity
  from_velocity : From  Commented=on  GotoTag=velocity
  from_velocity2 : From  Commented=on  GotoTag=velocity
  from_yaw_rate : From  Commented=on  GotoTag=yaw_rate
  from_yaw_rate2 : From  Commented=on  GotoTag=yaw_rate
  from_yaw_rate3 : From  Commented=on  GotoTag=yaw_rate
  radarDetections : adeye_lib/radarDetections  Commented=on  SystemSampleTime=-1
  wires:
  Camera_2/1(Camera_2) -> BMW_X5_SUV_1/9(Camera_2)
  Camera_tl/1(Camera_tl) -> BMW_X5_SUV_1/8(Camera_tl)
  Camera_1/1(Camera_1) -> BMW_X5_SUV_1/7(Camera_1)
  PointCloudSensor_4/1(PointCloudSensor_4) -> BMW_X5_SUV_1/6(PointCloudSensor_4)
  PointCloudSensor_3/1(PointCloudSensor_3) -> BMW_X5_SUV_1/5(PointCloudSensor_3)
  PointCloudSensor_2/1(PointCloudSensor_2) -> BMW_X5_SUV_1/4(PointCloudSensor_2)
  PointCloudSensor_1/1(PointCloudSensor_1) -> BMW_X5_SUV_1/3(PointCloudSensor_1)
  Radar_1/1(Radar_1) -> BMW_X5_SUV_1/2(Radar_1)
  Ford_Focus_Stationwagon_2/1(STATE_Ford_Focus_Stationwagon_2_bus) -> STATE_Ford_Focus_Stationwagon_2_bus/1(STATE_Ford_Focus_Stationwagon_2_bus)
  SELF_Ford_Focus_Stationwagon_2/1(SELF_Ford_Focus_Stationwagon_2) -> Ford_Focus_Stationwagon_2/1(SELF_Ford_Focus_Stationwagon_2)
  Child_Sitting_10/1(STATE_Child_Sitting_10_bus) -> STATE_Child_Sitting_10_bus/1(STATE_Child_Sitting_10_bus)
  SELF_Child_Sitting_10/1(SELF_Child_Sitting_10) -> Child_Sitting_10/1(SELF_Child_Sitting_10)
  Child_Sitting_10/2(VISUColorRegion_Upper_Body_Child_Sitting_10) -> VISUColorRegion_Upper_Body_Child_Sitting_10/1(VISUColorRegion_Upper_Body_Child_Sitting_10)
  Child_Sitting_10/3(VISUColorRegion_Lower_Body_Child_Sitting_10) -> VISUColorRegion_Lower_Body_Child_Sitting_10/1(VISUColorRegion_Lower_Body_Child_Sitting_10)
  Child_Sitting_10/4(VISUColorRegion_Shoes_Child_Sitting_10) -> VISUColorRegion_Shoes_Child_Sitting_10/1(VISUColorRegion_Shoes_Child_Sitting_10)
  Child_Leaning_1/1(STATE_Child_Leaning_1_bus) -> STATE_Child_Leaning_1_bus/1(STATE_Child_Leaning_1_bus)
  SELF_Child_Leaning_1/1(SELF_Child_Leaning_1) -> Child_Leaning_1/1(SELF_Child_Leaning_1)
  Child_Leaning_1/2(VISUColorRegion_Upper_Body_Child_Leaning_1) -> VISUColorRegion_Upper_Body_Child_Leaning_1/1(VISUColorRegion_Upper_Body_Child_Leaning_1)
  Child_Leaning_1/3(VISUColorRegion_Lower_Body_Child_Leaning_1) -> VISUColorRegion_Lower_Body_Child_Leaning_1/1(VISUColorRegion_Lower_Body_Child_Leaning_1)
  Child_Leaning_1/4(VISUColorRegion_Shoes_Child_Leaning_1) -> VISUColorRegion_Shoes_Child_Leaning_1/1(VISUColorRegion_Shoes_Child_Leaning_1)
  Child_Sitting_11/1(STATE_Child_Sitting_11_bus) -> STATE_Child_Sitting_11_bus/1(STATE_Child_Sitting_11_bus)
  SELF_Child_Sitting_11/1(SELF_Child_Sitting_11) -> Child_Sitting_11/1(SELF_Child_Sitting_11)
  Child_Sitting_11/2(VISUColorRegion_Upper_Body_Child_Sitting_11) -> VISUColorRegion_Upper_Body_Child_Sitting_11/1(VISUColorRegion_Upper_Body_Child_Sitting_11)
  Child_Sitting_11/3(VISUColorRegion_Lower_Body_Child_Sitting_11) -> VISUColorRegion_Lower_Body_Child_Sitting_11/1(VISUColorRegion_Lower_Body_Child_Sitting_11)
  Child_Sitting_11/4(VISUColorRegion_Shoes_Child_Sitting_11) -> VISUColorRegion_Shoes_Child_Sitting_11/1(VISUColorRegion_Shoes_Child_Sitting_11)
  Child_Sitting_12/1(STATE_Child_Sitting_12_bus) -> STATE_Child_Sitting_12_bus/1(STATE_Child_Sitting_12_bus)
  SELF_Child_Sitting_12/1(SELF_Child_Sitting_12) -> Child_Sitting_12/1(SELF_Child_Sitting_12)
  Child_Sitting_12/2(VISUColorRegion_Upper_Body_Child_Sitting_12) -> VISUColorRegion_Upper_Body_Child_Sitting_12/1(VISUColorRegion_Upper_Body_Child_Sitting_12)
  Child_Sitting_12/3(VISUColorRegion_Lower_Body_Child_Sitting_12) -> VISUColorRegion_Lower_Body_Child_Sitting_12/1(VISUColorRegion_Lower_Body_Child_Sitting_12)
  Child_Sitting_12/4(VISUColorRegion_Shoes_Child_Sitting_12) -> VISUColorRegion_Shoes_Child_Sitting_12/1(VISUColorRegion_Shoes_Child_Sitting_12)
  Child_Leaning_2/1(STATE_Child_Leaning_2_bus) -> STATE_Child_Leaning_2_bus/1(STATE_Child_Leaning_2_bus)
  SELF_Child_Leaning_2/1(SELF_Child_Leaning_2) -> Child_Leaning_2/1(SELF_Child_Leaning_2)
  Child_Leaning_2/2(VISUColorRegion_Upper_Body_Child_Leaning_2) -> VISUColorRegion_Upper_Body_Child_Leaning_2/1(VISUColorRegion_Upper_Body_Child_Leaning_2)
  Child_Leaning_2/3(VISUColorRegion_Lower_Body_Child_Leaning_2) -> VISUColorRegion_Lower_Body_Child_Leaning_2/1(VISUColorRegion_Lower_Body_Child_Leaning_2)
  Child_Leaning_2/4(VISUColorRegion_Shoes_Child_Leaning_2) -> VISUColorRegion_Shoes_Child_Leaning_2/1(VISUColorRegion_Shoes_Child_Leaning_2)
  Child_Leaning_3/1(STATE_Child_Leaning_3_bus) -> STATE_Child_Leaning_3_bus/1(STATE_Child_Leaning_3_bus)
  SELF_Child_Leaning_3/1(SELF_Child_Leaning_3) -> Child_Leaning_3/1(SELF_Child_Leaning_3)
  Child_Leaning_3/2(VISUColorRegion_Upper_Body_Child_Leaning_3) -> VISUColorRegion_Upper_Body_Child_Leaning_3/1(VISUColorRegion_Upper_Body_Child_Leaning_3)
  Child_Leaning_3/3(VISUColorRegion_Lower_Body_Child_Leaning_3) -> VISUColorRegion_Lower_Body_Child_Leaning_3/1(VISUColorRegion_Lower_Body_Child_Leaning_3)
  Child_Leaning_3/4(VISUColorRegion_Shoes_Child_Leaning_3) -> VISUColorRegion_Shoes_Child_Leaning_3/1(VISUColorRegion_Shoes_Child_Leaning_3)
  BMW_X5_SUV_1/1(STATE_BMW_X5_SUV_1_bus) -> STATE_BMW_X5_SUV_1_bus/1(STATE_BMW_X5_SUV_1_bus)
  SELF_BMW_X5_SUV_1/1(SELF_BMW_X5_SUV_1) -> BMW_X5_SUV_1/1(SELF_BMW_X5_SUV_1)
  Child_Regular_1/1(STATE_Child_Regular_1_bus) -> STATE_Child_Regular_1_bus/1(STATE_Child_Regular_1_bus)
  Child_Regular_1/2(ANIM_Child_Regular_1) -> ANIM_Child_Regular_1/1(ANIM_Child_Regular_1)
  SELF_Child_Regular_1/1(SELF_Child_Regular_1) -> Child_Regular_1/1(SELF_Child_Regular_1)
  Child_Regular_1/3(VISUColorRegion_Upper_Body_Child_Regular_1) -> VISUColorRegion_Upper_Body_Child_Regular_1/1(VISUColorRegion_Upper_Body_Child_Regular_1)
  Child_Regular_1/4(VISUColorRegion_Lower_Body_Child_Regular_1) -> VISUColorRegion_Lower_Body_Child_Regular_1/1(VISUColorRegion_Lower_Body_Child_Regular_1)
  Child_Regular_1/5(VISUColorRegion_Shoes_Child_Regular_1) -> VISUColorRegion_Shoes_Child_Regular_1/1(VISUColorRegion_Shoes_Child_Regular_1)
  Nissan_Cabstar_Boxtruck_1/1(STATE_Nissan_Cabstar_Boxtruck_1_bus) -> STATE_Nissan_Cabstar_Boxtruck_1_bus/1(STATE_Nissan_Cabstar_Boxtruck_1_bus)
  SELF_Nissan_Cabstar_Boxtruck_1/1(SELF_Nissan_Cabstar_Boxtruck_1) -> Nissan_Cabstar_Boxtruck_1/1(SELF_Nissan_Cabstar_Boxtruck_1)
  Female_Regular_1/1(STATE_Female_Regular_1_bus) -> STATE_Female_Regular_1_bus/1(STATE_Female_Regular_1_bus)
  Female_Regular_1/2(ANIM_Female_Regular_1) -> ANIM_Female_Regular_1/1(ANIM_Female_Regular_1)
  SELF_Female_Regular_1/1(SELF_Female_Regular_1) -> Female_Regular_1/1(SELF_Female_Regular_1)
  Female_Regular_1/3(VISUColorRegion_Upper_Body_Female_Regular_1) -> VISUColorRegion_Upper_Body_Female_Regular_1/1(VISUColorRegion_Upper_Body_Female_Regular_1)
  Female_Regular_1/4(VISUColorRegion_Lower_Body_Female_Regular_1) -> VISUColorRegion_Lower_Body_Female_Regular_1/1(VISUColorRegion_Lower_Body_Female_Regular_1)
  Female_Regular_1/5(VISUColorRegion_Shoes_Female_Regular_1) -> VISUColorRegion_Shoes_Female_Regular_1/1(VISUColorRegion_Shoes_Female_Regular_1)
  RoadsideLight_NL_1/1(RoadsideLight_NL_1_Red) -> RoadsideLight_NL_1_Red/1(RoadsideLight_NL_1_Red)
  RoadsideLight_NL_1/2(RoadsideLight_NL_1_Orange) -> RoadsideLight_NL_1_Orange/1(RoadsideLight_NL_1_Orange)
  RoadsideLight_NL_1/3(RoadsideLight_NL_1_Green) -> RoadsideLight_NL_1_Green/1(RoadsideLight_NL_1_Green)
  from_velicty3/1 -> ROS Send IMU/5
  GoalOrientW/1 -> ROS Send Goal/4
  from_lidar3/1 -> ROS Send Lidar/3
  EnableSendFeatures/1 -> ROS Send Simulink State/Enable
  from_camera2_b/1 -> ROS Send Camera 2/3
  Localization/1 -> ROS Send Simulink State/4
  Sensing/1 -> ROS Send Simulink State/3
  from_velocity/1 -> ROS Send Velocity/1
  EnableSendCameraTL/1 -> ROS Send Camera TL/Enable
  from_roty/1 -> ROS Send IMU/2
  GoalPoseZ/1 -> ROS Send Goal/3
  from_camera_tl_r/1 -> ROS Send Camera TL/1
  Map/1 -> ROS Send Simulink State/2
  from_base_link_pose2/1 -> ROS Send Odometry/1
  EnableSendCamera1/1 -> ROS Send Camera/Enable
  EnableSendIMU/1 -> ROS Send IMU/Enable
  from_camera1_g/1 -> ROS Send Camera/2
  from_yaw_rate2/1 -> ROS Send Odometry/3
  from_yaw_rate3/1 -> ROS Send IMU/4
  Switch/1 -> ROS Send Simulink State/9
  GoalOrientZ/1 -> ROS Send Goal/7
  from_rotx/1 -> ROS Send IMU/1
  from_camera_tl_g/1 -> ROS Send Camera TL/2
  Ssmp/1 -> ROS Send Simulink State/10
  MotionPlanning/1 -> ROS Send Simulink State/8
  from_lidar4/1 -> ROS Send Lidar/4
  from_lidar2/1 -> ROS Send Lidar/2
  from_rotz/1 -> ROS Send IMU/3
  EnableSendGNSS/1 -> ROS Send GNSS/Enable
  from_lidar1/1 -> ROS Send Lidar/1
  EnableSendRadar/1 -> radarDetections/Enable
  from_radar_theta/1 -> radarDetections/2
  Fault/1 -> ROS send RCV states/3
  EnableSendSwitch/1 -> ROS Send Switch Command/Enable
  from_camera2_g/1 -> ROS Send Camera 2/2
  from_camera1_r/1 -> ROS Send Camera/1
  Detection/1 -> ROS Send Simulink State/6
  Rviz/1 -> ROS Send Simulink State/11
  EnableSendClock/1 -> ROS Send Clock/Enable
  MissionPlanning/1 -> ROS Send Simulink State/7
  GoalPoseY/1 -> ROS Send Goal/2
  Activation request/1 -> ROS send RCV states/2
  EnableSendCamera2/1 -> ROS Send Camera 2/Enable
  FakeLocalization/1 -> ROS Send Simulink State/5
  from_gnss_pose/1 -> ROS Send GNSS/1
  Recording/1 -> ROS Send Simulink State/1
  Initial checks/1 -> ROS send RCV states/1
  EnableSendOdometry/1 -> ROS Send Odometry/Enable
  from_yaw_rate/1 -> ROS Send Velocity/2
  SwitchCommand/1 -> ROS Send Switch Command/1
  GoalOrientY/1 -> ROS Send Goal/6
  from_radar_targetID/1 -> radarDetections/4
  from_camera2_r/1 -> ROS Send Camera 2/1
  EnableSendVelocity/1 -> ROS Send Velocity/Enable
  from_radar_phi/1 -> radarDetections/3
  Clock2/1 -> Relational Operator1/1
  from_camera1_b/1 -> ROS Send Camera/3
  EnableSendLidar/1 -> ROS Send Lidar/Enable
  Relational Operator1/1 -> ROS Send Goal/Enable
  Clock/1 -> ROS Send Clock/1
  GoalOrientX/1 -> ROS Send Goal/5
  Constant27/1 -> Relational Operator1/2
  from_radar_range/1 -> radarDetections/1
  from_camera_tl_b/1 -> ROS Send Camera TL/3
  GoalPoseX/1 -> ROS Send Goal/1
  from_velocity2/1 -> ROS Send Odometry/2
